simulink model "pll_21"  (Simulink 2.20)
settings: Solver=ode45  StartTime=0.0  StopTime=10.0  RelTol=1e-3  AbsTol=1e-6
values from neighbouring files (symbols this model uses):
  f0 = 500    [chirp_1.m]    (also in costas1f.m = pf0; op_freq.m = 15; pll_5f.m = f01)
  kvco = pkvco    [costas1f.m]    (also in pll_5f.m = kvco1)
  tau = ptau    [costas1f.m]    (also in op_freq.m = 0.0106103295395; pll_5f.m = tau1)
settings Model: ConsistencyChecking=off  RTWPlaceOutputsASAP=off

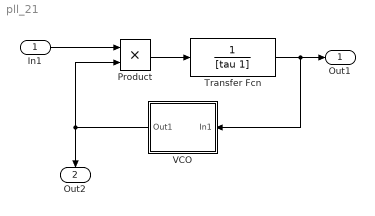
== system pll_21 ==
  In1 : Inport  Port=1  PortWidth=-1  SampleTime=-1
  Product : Product  Inputs=2
  Transfer Fcn : TransferFcn  Numerator=[1]  Denominator=[tau 1]
  VCO : Subsystem  Orientation=left
  Out1 : Outport  Port=1
  Out2 : Outport  Orientation=down  Port=2
  wires:
  In1/1 -> Product/1
  Product/1 -> Transfer Fcn/1
  Transfer Fcn/1 -> Out1/1, VCO/1(In1)
  VCO/1(Out1) -> Product/2, Out2/1

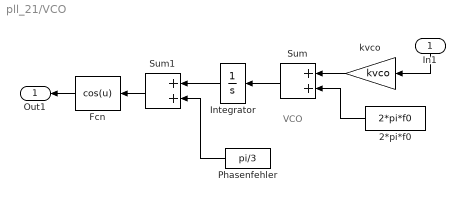
== system pll_21/VCO ==
  note: VCO
  In1 : Inport  Orientation=down  Port=1  PortWidth=-1  SampleTime=-1
  2*pi*f0 : Constant  Orientation=left  Value=2*pi*f0
  Fcn : Fcn  Orientation=left  Expr=cos(u)
  Integrator : Integrator  Orientation=left  ExternalReset=none  InitialConditionSource=internal  InitialCondition=0  LimitOutput=off  UpperSaturationLimit=inf  LowerSaturationLimit=-inf  ShowSaturationPort=off  ShowStatePort=off  AbsoluteTolerance=auto
  Phasenfehler : Constant  Orientation=left  Value=pi/3
  Sum : Sum  Orientation=left  Inputs=++
  Sum1 : Sum  Orientation=left  Inputs=++
  kvco : Gain  Orientation=left  Gain=kvco
  Out1 : Outport  Orientation=left  Port=1  InitialOutput=0
  wires:
  Sum/1 -> Integrator/1
  2*pi*f0/1 -> Sum/2
  kvco/1 -> Sum/1
  In1/1 -> kvco/1
  Sum1/1 -> Fcn/1
  Integrator/1 -> Sum1/1
  Phasenfehler/1 -> Sum1/2
  Fcn/1 -> Out1/1
